simulink model "massspringdamping"  (R2023a)
settings: Solver=VariableStepAuto  StartTime=0.0  StopTime=10.0  RelTol=1e-3
settings Model: Creator=Aditya Singh Yadav  LastModifiedBy=Aditya Singh Yadav

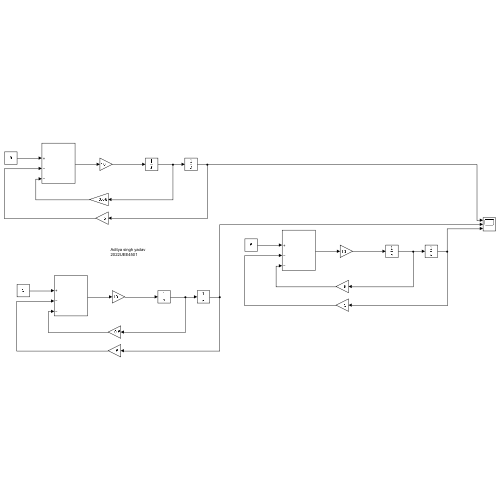
[thumbnail: Simulink's stored preview of the top-level diagram]
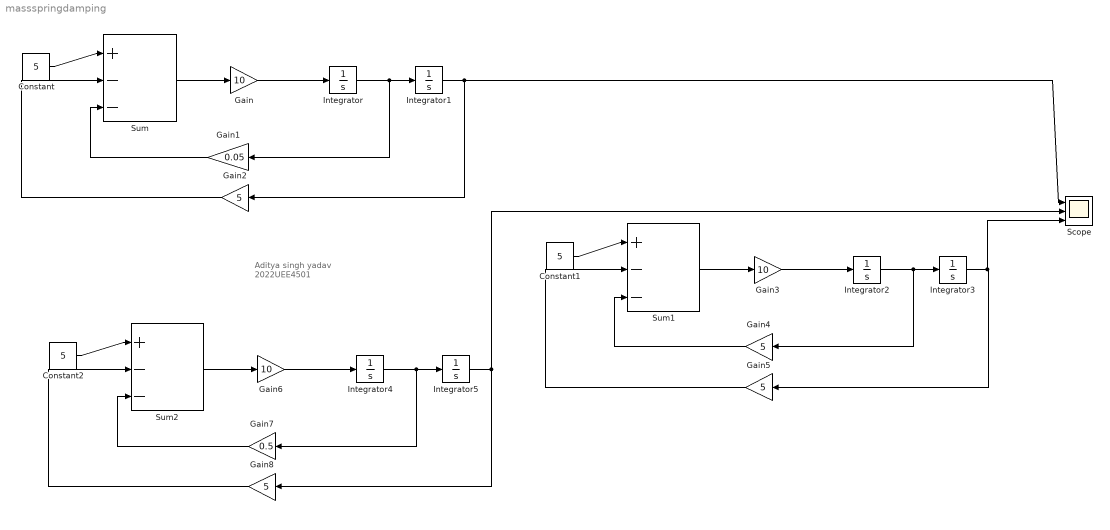
== system massspringdamping ==
  note: Aditya singh yadav
      | 2022UEE4501
  Constant : Constant  Value=5
  Constant1 : Constant  Value=5
  Constant2 : Constant  Value=5
  Gain : Gain  Gain=10
  Gain1 : Gain  Gain=0.05
  Gain{2,4..5,8} (4 alike) : Gain  Gain=5
  Gain3 : Gain  Gain=10
  Gain6 : Gain  Gain=10
  Gain7 : Gain  Gain=0.5
  Integrator{,1..5} (6 alike) : Integrator
  Scope : Scope  NumInputPorts=3
  Sum : Sum  Inputs=|+--
  Sum1 : Sum  Inputs=|+--
  Sum2 : Sum  Inputs=|+--
  wires:
  Gain2/1 -> Sum/2
  Integrator1/1 -> Gain2/1, Scope/1
  Gain/1 -> Integrator/1
  Gain1/1 -> Sum/3
  Constant/1 -> Sum/1
  Sum/1 -> Gain/1
  Integrator/1 -> Gain1/1, Integrator1/1
  Gain5/1 -> Sum1/2
  Integrator3/1 -> Scope/3, Gain5/1
  Gain3/1 -> Integrator2/1
  Gain4/1 -> Sum1/3
  Constant1/1 -> Sum1/1
  Sum1/1 -> Gain3/1
  Integrator2/1 -> Gain4/1, Integrator3/1
  Gain8/1 -> Sum2/2
  Integrator5/1 -> Scope/2, Gain8/1
  Gain6/1 -> Integrator4/1
  Gain7/1 -> Sum2/3
  Constant2/1 -> Sum2/1
  Sum2/1 -> Gain6/1
  Integrator4/1 -> Gain7/1, Integrator5/1
